simulink model "PO_Boost_sari"  (R2016a)
settings: Solver=VariableStepAuto  StartTime=0.0  StopTime=10.0  RelTol=1e-3
libraries: powerlib x13, powerlib_extras x2, simulink x1
settings Model: Creator=AIMS  LastModifiedBy=AIMS

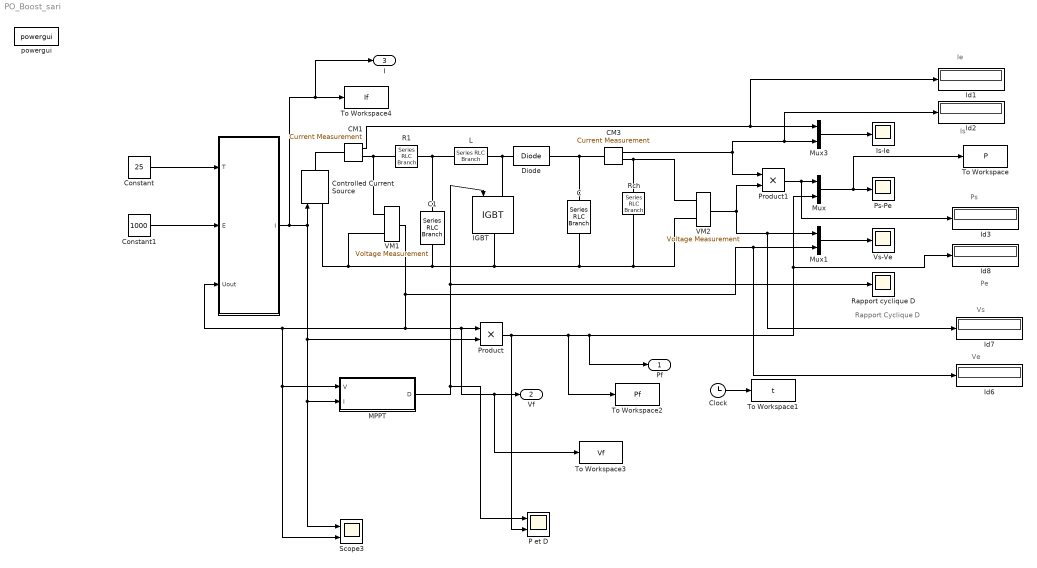
== system PO_Boost_sari ==
  note: Rapport Cyclique D
  note: Pe
  note: Ps
  note: Is
  note: Ie
  note: Ve
  note: Vs
  " " : Subsystem
  C : powerlib/Elements/Series RLC Branch  LConnTagsString=__new0  RConnTagsString=__new0  BranchType=C  Resistance=0.01  Inductance=1.0  SetiL0=off  InitialCurrent=0  Capacitance=2e-3  Setx0=off  InitialVoltage=200  Measurements=None
  C1 : powerlib/Elements/Series RLC Branch  LConnTagsString=__new0  RConnTagsString=__new0  BranchType=C  Resistance=0.01  Inductance=1.0  SetiL0=off  InitialCurrent=0  Capacitance=2e-3  Setx0=off  InitialVoltage=0  Measurements=None
  CM1 : powerlib/Measurements/Current Measurement  Tag=PoWeRsYsTeMmEaSuReMeNt  PhasorSimulation=off  OutputType=Magnitude  PSBequivalent=0
  CM3 : powerlib/Measurements/Current Measurement  Tag=PoWeRsYsTeMmEaSuReMeNt  PhasorSimulation=off  OutputType=Magnitude  PSBequivalent=0
  Clock : Clock
  Constant : Constant  Value=25
  Constant1 : Constant  Value=1000
  Controlled Current Source : powerlib/Electrical Sources/Controlled Current Source  Initialize=on  Source_Type=AC  Amplitude=0  Phase=0  Frequency=0  Measurements=None
  Diode : powerlib/Power Electronics/Diode  Ron=0.001  Lon=0  Vf=0.8  IC=0  UseSnubber=off  Rs=500  Cs=250e-9  Measurements=off
  IGBT : powerlib/Power Electronics/IGBT  Ron=0.001  Lon=0  Vf=1  Tf=1e-6  Tt=2e-6  IC=0  Rs=1e5  Cs=inf  Measurements=off
  Id{1..3,6..8} (6 alike) : Display
  Is-Ie : Scope
  L : powerlib/Elements/Series RLC Branch  LConnTagsString=__new0  RConnTagsString=__new0  BranchType=L  Resistance=1.0  Inductance=0.002  SetiL0=off  InitialCurrent=0  Capacitance=1.0  Setx0=off  InitialVoltage=0  Measurements=None
  MPPT : Subsystem
  Mux : Mux  Inputs=2
  Mux1 : Mux  Inputs=2
  Mux3 : Mux  Inputs=2
  "P et D " : Scope  NumInputPorts=2
  Product : Product  RndMeth=Zero
  Product1 : Product  RndMeth=Zero
  Ps-Pe : Scope
  R1 : powerlib/Elements/Series RLC Branch  LConnTagsString=__new0  RConnTagsString=__new0  BranchType=R  Resistance=1  Inductance=1.0  SetiL0=off  InitialCurrent=0  Capacitance=1.0  Setx0=off  InitialVoltage=0  Measurements=None
  Rapport cyclique D : Scope
  Rch : powerlib/Elements/Series RLC Branch  LConnTagsString=__new0  RConnTagsString=__new0  BranchType=R  Resistance=10  Inductance=1.0  SetiL0=off  InitialCurrent=0  Capacitance=1.0  Setx0=off  InitialVoltage=0  Measurements=None
  Scope3 : Scope  NumInputPorts=2
  To Workspace : ToWorkspace  VariableName=P  SampleTime=-1
  To Workspace1 : ToWorkspace  VariableName=t  SampleTime=-1
  To Workspace2 : ToWorkspace  VariableName=Pf  SampleTime=-1
  To Workspace3 : ToWorkspace  VariableName=Vf  SampleTime=-1
  To Workspace4 : ToWorkspace  VariableName=If  SampleTime=-1
  VM1 : powerlib/Measurements/Voltage Measurement  Tag=PoWeRsYsTeMmEaSuReMeNt  PhasorSimulation=off  OutputType=Magnitude  PSBequivalent=0
  VM2 : powerlib/Measurements/Voltage Measurement  Tag=PoWeRsYsTeMmEaSuReMeNt  PhasorSimulation=off  OutputType=Magnitude  PSBequivalent=0
  Vs-Ve : Scope
  powergui : powerlib/powergui  SimulationMode=Continuous  SolverType=Tustin  SampleTime=50e-6  frequency=60  SPID=off  DisableSnubberDevices=off  DisableRonSwitches=off  DisableVfSwitches=off  SwTol=0  DisplayEquations=off  Interpol=off  ExternalGateDelay=off  methode=off  Ts=0  FunctionMessages=off  echomessages=off  HookPort=off  EnableUseOfTLC=off  x0status=blocks  frequencyindice=0  Pbase=100e6  ErrMax=1e-4  Iterations=50  UnitsV=kV  UnitsW=MW  buscounter=0  RestoreLinks=warning  ResistiveCurrentMeasurement=off  Frange=[0:2:500]  Ylog=off  Xlog=on  ShowGrid=off  save=off  variable=ZData  structure=mmmm  ZoomFFT=off  StartTime=0.0  cycles=1  DisplayStyle=1  fundamental=60  FreqAxis=off  MaxFrequency=1000  frequencyindicesteady=1  RmsSteady=1  display=off
  Pf : Outport
  Vf : Outport  Port=2
  "I  " : Outport  Port=3
  wires:
  " "/1(I) -> Controlled Current Source/1, Product/2, Scope3/1, MPPT/2(I), To Workspace4/1, "I  "/1
  CM3/1 -> Id2/1, Mux3/2, Product1/1
  VM2/1 -> Id7/1, Mux1/1, Product1/2
  Product1/1 -> Id3/1, Mux/1
  VM1/1 -> Id6/1, Mux1/2, " "/3(Uout), Scope3/2, MPPT/1(V), Product/1, Vf/1, To Workspace3/1
  Mux/1 -> Ps-Pe/1, To Workspace/1
  Mux1/1 -> Vs-Ve/1
  CM1/1 -> Id1/1, Mux3/1
  Mux3/1 -> Is-Ie/1
  MPPT/1(D) -> "P et D "/1, IGBT/1, Rapport cyclique D/1
  Clock/1 -> To Workspace1/1
  Constant1/1 -> " "/2(E)
  Constant/1 -> " "/1(T)
  Product/1 -> Id8/1, Mux/2, Pf/1, To Workspace2/1, "P et D "/2
  connections:
  C/RConn1 -- Controlled Current Source/LConn1 -- VM1/LConn2 -- C1/RConn1 -- IGBT/RConn1 -- VM2/LConn2 -- Rch/RConn1
  CM3/LConn1 -- Diode/RConn1 -- C/LConn1
  L/RConn1 -- Diode/LConn1 -- IGBT/LConn1
  Rch/LConn1 -- CM3/RConn1 -- VM2/LConn1
  R1/RConn1 -- VM1/LConn1 -- CM1/RConn1
  L/LConn1 -- R1/LConn1 -- C1/LConn1
  Controlled Current Source/RConn1 -- CM1/LConn1

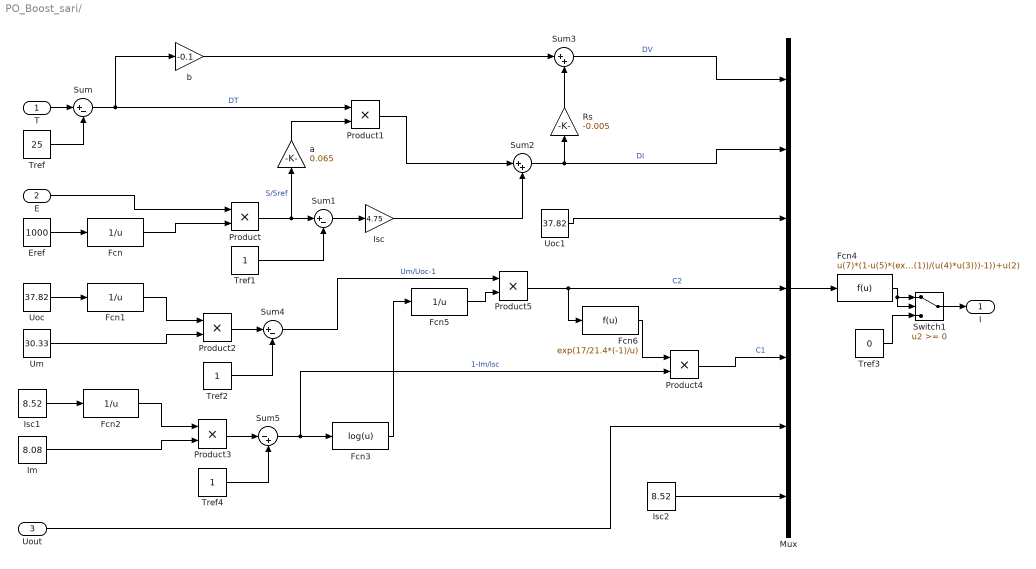
== system PO_Boost_sari/  ==
  T : Inport
  E : Inport  Port=2
  Uout : Inport  Port=3
  Eref : Constant  Value=1000
  Fcn{,1..2,5} (4 alike) : Fcn  Expr=1/u
  Fcn3 : Fcn  Expr=log(u)
  Fcn4 : Fcn  Expr=u(7)*(1-u(5)*(exp((u(6)-u(1))/(u(4)*u(3)))-1))+u(2)
  Fcn6 : Fcn  Expr=exp(17/21.4*(-1)/u)
  Im : Constant  Value=8.08
  Isc : Gain  Gain=4.75
  Isc1 : Constant  Value=8.52
  Isc2 : Constant  Value=8.52
  Mux : Mux  Inputs=7
  Product{,1..5} (6 alike) : Product  RndMeth=Zero
  Rs : Gain  Gain=-0.005
  Sum : Sum  Inputs=|+-
  Sum1 : Sum  Inputs=|+-
  Sum2 : Sum  Inputs=|++
  Sum3 : Sum  Inputs=|++
  Sum4 : Sum  Inputs=|+-
  Sum5 : Sum  Inputs=|-+
  Switch1 : Switch
  Tref : Constant  Value=25
  Tref1 : Constant
  Tref2 : Constant
  Tref3 : Constant  Value=0
  Tref4 : Constant
  Um : Constant  Value=30.33
  Uoc : Constant  Value=37.82
  Uoc1 : Constant  Value=37.82
  a : Gain  Gain=0.065
  b : Gain  Gain=-0.1
  I : Outport
  wires:
  T/1 -> Sum/1
  Tref/1 -> Sum/2
  Sum/1 -> Product1/1, b/1  "DT"
  Eref/1 -> Fcn/1
  Fcn/1 -> Product/2
  E/1 -> Product/1
  Product/1 -> Sum1/1, a/1  "S/Sref"
  Tref1/1 -> Sum1/2
  Sum1/1 -> Isc/1
  a/1 -> Product1/2
  Product1/1 -> Sum2/1
  Isc/1 -> Sum2/2
  Sum2/1 -> Rs/1, Mux/2  "DI"
  b/1 -> Sum3/1
  Rs/1 -> Sum3/2
  Sum3/1 -> Mux/1  "DV"
  Uoc/1 -> Fcn1/1
  Fcn1/1 -> Product2/1
  Um/1 -> Product2/2
  Product2/1 -> Sum4/1
  Tref2/1 -> Sum4/2
  Isc1/1 -> Fcn2/1
  Fcn2/1 -> Product3/1
  Im/1 -> Product3/2
  Product3/1 -> Sum5/1
  Tref4/1 -> Sum5/2
  Sum5/1 -> Fcn3/1, Product4/2  "1-Im/Isc"
  Mux/1 -> Fcn4/1
  Uoc1/1 -> Mux/3
  Uout/1 -> Mux/6
  Isc2/1 -> Mux/7
  Product5/1 -> Mux/4, Fcn6/1  "C2"
  Sum4/1 -> Product5/1  "Um/Uoc-1"
  Fcn3/1 -> Fcn5/1
  Fcn5/1 -> Product5/2
  Fcn6/1 -> Product4/1
  Product4/1 -> Mux/5  "C1"
  Tref3/1 -> Switch1/3
  Fcn4/1 -> Switch1/1, Switch1/2
  Switch1/1 -> I/1

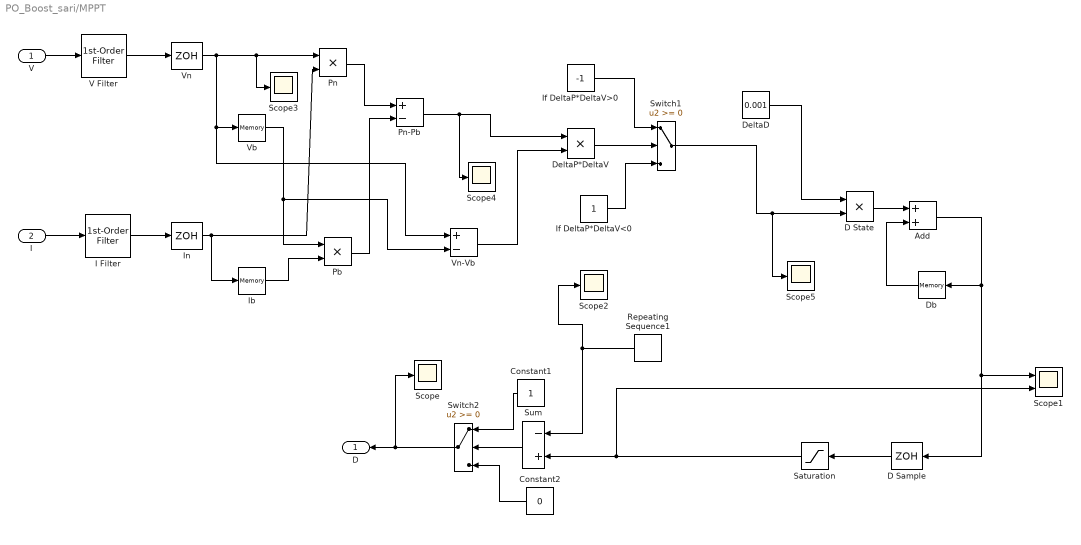
== system PO_Boost_sari/MPPT ==
  V : Inport
  I : Inport  Port=2
  Add : Sum
  Constant1 : Constant  SampleTime=-1
  Constant2 : Constant  Value=0  SampleTime=-1
  D Sample : ZeroOrderHold  SampleTime=1e-4
  D State : Product  RndMeth=Zero
  Db : Memory  InheritSampleTime=on  LinearizeAsDelay=on
  DeltaD : Constant  Value=0.001
  DeltaP*DeltaV : Product  RndMeth=Zero
  I Filter : powerlib_extras/Control  Blocks/1st-Order  Filter  FilterType=Lowpass  Tc=1e-3  Initialize=off  Vac_Init=[0.8 -25 60]  Vdc_Init=-0.4  PlotResponse=off  param1=[1 500 1]
  Ib : Memory  InheritSampleTime=on  LinearizeAsDelay=on
  If DeltaP*DeltaV<0 : Constant
  If DeltaP*DeltaV>0 : Constant  Value=-1
  In : ZeroOrderHold  SampleTime=1e-4
  Pb : Product  RndMeth=Zero
  Pn : Product  RndMeth=Zero
  Pn-Pb : Sum  Inputs=+-
  Repeating Sequence1 : simulink/Sources/Repeating Sequence  rep_seq_t=[0 4e-3 4e-2]  rep_seq_y=[0 1 0]
  Saturation : Saturate  UpperLimit=0.8  LowerLimit=0
  Scope{,2..5} (5 alike) : Scope
  Scope1 : Scope  NumInputPorts=2
  Sum : Sum  Inputs=-+  SaturateOnIntegerOverflow=on
  Switch1 : Switch
  Switch2 : Switch
  V Filter : powerlib_extras/Control  Blocks/1st-Order  Filter  FilterType=Lowpass  Tc=1e-3  Initialize=off  Vac_Init=[0.8 -25 60]  Vdc_Init=-0.4  PlotResponse=off  param1=[1 500 1]
  Vb : Memory  InheritSampleTime=on  LinearizeAsDelay=on
  Vn : ZeroOrderHold  SampleTime=1e-4
  Vn-Vb : Sum  Inputs=+-
  D : Outport
  wires:
  V/1 -> V Filter/1
  I/1 -> I Filter/1
  V Filter/1 -> Vn/1
  I Filter/1 -> In/1
  In/1 -> Ib/1, Pn/2
  Vn/1 -> Scope3/1, Pn/1, Vb/1, Vn-Vb/1
  Ib/1 -> Pb/2
  Vb/1 -> Pb/1, Vn-Vb/2
  Pn/1 -> Pn-Pb/1
  Pb/1 -> Pn-Pb/2
  D State/1 -> Add/1
  Constant2/1 -> Switch2/3
  Constant1/1 -> Switch2/1
  Sum/1 -> Switch2/2
  Repeating Sequence1/1 -> Sum/1, Scope2/1
  Add/1 -> Db/1, D Sample/1, Scope1/1
  Switch2/1 -> Scope/1, D/1
  Db/1 -> Add/2
  D Sample/1 -> Saturation/1
  Pn-Pb/1 -> Scope4/1, DeltaP*DeltaV/1
  Vn-Vb/1 -> DeltaP*DeltaV/2
  DeltaP*DeltaV/1 -> Switch1/2
  If DeltaP*DeltaV>0/1 -> Switch1/1
  If DeltaP*DeltaV<0/1 -> Switch1/3
  Switch1/1 -> Scope5/1, D State/2
  DeltaD/1 -> D State/1
  Saturation/1 -> Sum/2, Scope1/2
